simulink model "Q1"  (R2022a)
settings: Solver=FixedStepDiscrete  StartTime=0.0  StopTime=1  FixedStep=Ts  RelTol=1e-3
InitFcn:
  | Ts=50e-6;
  | 
  | % Rectifier AC side :
  | VLL_nom_R = 500e3; % V
  | Fnom_R = 60;           % Hz
  | 
  | % Inverter AC side :
  | VLL_nom_I = 345e3; % V
  | Fnom_I = 50;           % Hz
  | 
  | % DC :
  | Vdc_nom = 500e3;   % V
  | Idc_nom  = 2000;     % A
undefined symbols (not defined in the file or in its folder): D1, Delta, lagging, pulse
libraries: powerlib_extras x6, spsThreePhaseHarmonicFilterLib x6, spsImpedanceMeasurementLib x4, spsUniversalBridgeLib x4, spsThreePhaseSourceLib x2, spsSeriesRLCBranchLib x2, spsThreePhaseParallelRLCBranchLib x2, spsThreePhaseVIMeasurementLib x2, spsGroundLib x2, spsThreePhaseTransformerThreeWindingsLib x2, spsPLL3phLib x2, spsPulseGeneratorThyristor12PulseLib x2
settings Model: Creator=BhAsKaR  LastModifiedBy=ds
settings SolverCC: AlgebraicLoopSolver=TrustRegion
settings DataIOCC: SaveTime=off  ReturnWorkspaceOutputs=off
settings OptimizationCC: DefaultParameterBehavior=Inlined  EnhancedBackFolding=on  PassReuseOutputArgsAs=Individual arguments  ZeroExternalMemoryAtStartup=off  ZeroInternalMemoryAtStartup=off  OptimizeBlockOrder=speed  DifferentSizesBufferReuse=on  OptimizationCustomize=off  EfficientTunableParamExpr=on
settings DebuggingCC: ParameterTunabilityLossMsg=error  UnconnectedInputMsg=warning  UnconnectedOutputMsg=warning  SFMachineParentedDataDiag=warning
settings SFSimCC: MATLABDynamicMemAlloc=off
settings RTWCC: SystemTargetFile=ert.tlc  TemplateMakefile=ert_default_tmf
settings CodeAppCC: ForceParamTrailComments=on  IgnoreCustomStorageClasses=off  OperatorAnnotations=on  SimulinkDataObjDesc=on  SFDataObjDesc=on  InsertBlockDesc=on
settings ERTTargetCC: TargetLangStandard=C99 (ISO)  GenerateSampleERTMain=on  InlinedParameterPlacement=NonHierarchical  ERTCustomFileTemplate=example_file_process.tlc

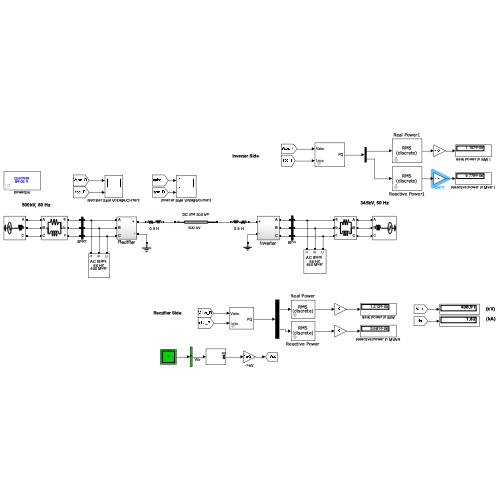
[thumbnail: Simulink's stored preview of the top-level diagram]
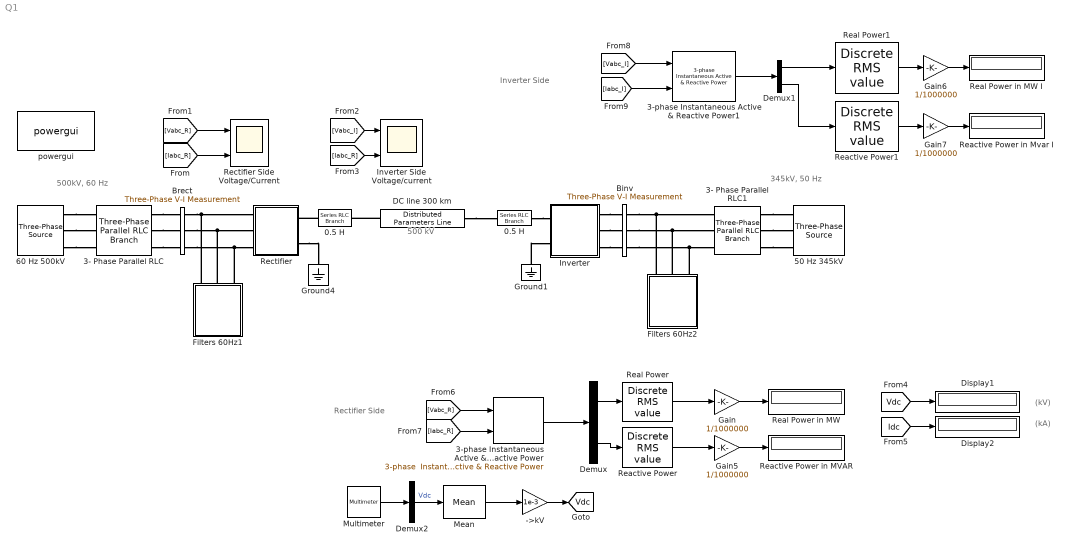
== system Q1 ==
  note: 500 kV
  note: 500kV, 60 Hz
  note: 345kV, 50 Hz
  note: (kV)
  note: Rectifier Side
  note: Inverter Side
  note: (kA)
  " 50 Hz 345kV  " : spsThreePhaseSourceLib/Three-Phase Source  InternalConnection=Yg  VoltagePhases=off  Voltage=VLL_nom_I  PhaseAngle=0  Voltage_phases=[25e3 25e3 25e3]/sqrt(3)  PhaseAngles_phases=[0 -120 +120]  Frequency=Fnom_I  NonIdealSource=on  SpecifyImpedance=off  Resistance=0  Inductance=28.0e-3  ShortCircuitLevel=0  BaseVoltage=0  XRratio=0  BusType=swing  Pref=0  Qref=0  Prefabc=[10e3, 10e3, 10e3]  Qrefabc=[0, 0, 0]  Qmin=-inf  Qmax=inf
  " 60 Hz 500kV" : spsThreePhaseSourceLib/Three-Phase Source  InternalConnection=Yg  VoltagePhases=off  Voltage=VLL_nom_R  PhaseAngle=0  Voltage_phases=[25e3 25e3 25e3]/sqrt(3)  PhaseAngles_phases=[0 -120 +120]  Frequency=Fnom_R  NonIdealSource=on  SpecifyImpedance=off  Resistance=0  Inductance=98.03e-3  ShortCircuitLevel=0  BaseVoltage=0  XRratio=0  BusType=swing  Pref=0  Qref=0  Prefabc=[10e3, 10e3, 10e3]  Qrefabc=[0, 0, 0]  Qmin=-inf  Qmax=inf
  ->kV : Gain  Gain=1e-3  SaturateOnIntegerOverflow=on  OutDataTypeStr=Inherit: Same as input  ParamDataTypeStr=Inherit: Same as input
  0.5 H : spsSeriesRLCBranchLib/Series RLC Branch  LConnTagsString=__new0  RConnTagsString=__new0  BranchType=RL  Resistance=1  Inductance=0.5  SetiL0=off  InitialCurrent=0  Capacitance=1.0  Setx0=off  InitialVoltage=0  Measurements=Branch voltage and current
  "0.5 H " : spsSeriesRLCBranchLib/Series RLC Branch  LConnTagsString=__new0  RConnTagsString=__new0  BranchType=RL  Resistance=1  Inductance=0.5  SetiL0=off  InitialCurrent=0  Capacitance=1.0  Setx0=off  InitialVoltage=0  Measurements=Branch voltage and current
  3- Phase Parallel RLC : spsThreePhaseParallelRLCBranchLib/Three-Phase Parallel RLC Branch  LConnTagsString=A|B|C  RConnTagsString=A|B|C  BranchType=RL  Resistance=26.07  Inductance=48.86e-3  Capacitance=1.0  Measurements=None
      settings: SourceProductBaseCode=PS
  3- Phase Parallel RLC1 : spsThreePhaseParallelRLCBranchLib/Three-Phase Parallel RLC Branch  LConnTagsString=A|B|C  RConnTagsString=A|B|C  BranchType=RL  Resistance=6.205  Inductance=13.96e-3  Capacitance=1.0  Measurements=None
      settings: SourceProductBaseCode=PS
  3-phase Instantaneous Active & Reactive Power : powerlib_extras/Measurements/3-phase  Instantaneous  Active & Reactive Power
      settings: SourceProductBaseCode=PS
  3-phase Instantaneous Active & Reactive Power1 : powerlib_extras/Measurements/3-phase  Instantaneous  Active & Reactive Power
      settings: SourceProductBaseCode=PS
  Binv : spsThreePhaseVIMeasurementLib/Three-Phase V-I Measurement  VoltageMeasurement=phase-to-ground  SetLabelV=on  LabelV=Vabc_I  Vpu=on  VpuLL=off  CurrentMeasurement=yes  SetLabelI=on  LabelI=Iabc_I  Ipu=on  Pbase=100e6  Vbase=345e3  OutputType=Magnitude  PhasorSimulation=off  PSBequivalent=0
  Brect : spsThreePhaseVIMeasurementLib/Three-Phase V-I Measurement  VoltageMeasurement=phase-to-ground  SetLabelV=on  LabelV=Vabc_R  Vpu=on  VpuLL=off  CurrentMeasurement=yes  SetLabelI=on  LabelI=Iabc_R  Ipu=on  Pbase=100e6  Vbase=500e3  OutputType=Magnitude  PhasorSimulation=off  PSBequivalent=0
  DC line 300 km : spsDistributedParametersLineLib/Distributed Parameters Line  Phases=1  Length=300  Frequency=60  Resistance=0.015  Inductance=0.792e-3  Capacitance=14.4e-9  x1=[-0.00105 -5.9657325618739e-12;-0.001 -5.74588371812075e-12;-0.00095 -5.52535227515782e-12;-0.0009 -5.30421024315457e-12;-0.00085 -5.08252951550024e-12;-0.0008 -4.86038184490804e-12;-0.00075 -4.63783881965118e-12;-0.0007 -4.41497183993891e-12;-0.00065 -4.19185209444034e-12;-0.0006 -3.96855053696411e-12;-0.00055 -3.74513786330158e-12;-0.0005 -3.52168448824124e-12;-0.00045 -3.29826052276211e-12;-0.0004 -3.07493575141354e-12;-0.00035 -2.85177960988905e-12;-0.0003 -2.62886116280138e-12;-0.00025 -2.40624908166623e-12;-0.0002 -2.18401162310181e-12;-0.00015 -1.96221660725129e-12;-0.0001 -1.74093139643523e-12;-5e-05 -1.52022287404077e-12]  x2=[-0.00105 -4.80956103183517e-12;-0.001 -4.57813962792348e-12;-0.00095 -4.34637866135639e-12;-0.0009 -4.11435439321598e-12;-0.00085 -3.88214286207982e-12;-0.0008 -3.64981985858362e-12;-0.00075 -3.41746090014951e-12;-0.0007 -3.18514120588852e-12;-0.00065 -2.95293567168596e-12;-0.0006 -2.72091884547773e-12;-0.00055 -2.48916490272637e-12;-0.0005 -2.2577476221045e-12;-0.00045 -2.0267403613944e-12;-0.0004 -1.79621603361121e-12;-0.00035 -1.56624708335811e-12;-0.0003 -1.33690546342109e-12;-0.00025 -1.10826261161117e-12;-0.0002 -8.80389427861601e-13;-0.00015 -6.53356251587666e-13;-0.0001 -4.27232839316443e-13;-5e-05 -2.02088342593868e-13]  x3=[-0.00105 -4.02613211172553e-14;-0.001 -3.91158507623226e-14;-0.00095 -3.79621871436524e-14;-0.0009 -3.6800712983211e-14;-0.00085 -3.56318123772384e-14;-0.0008 -3.44558706668299e-14;-0.00075 -3.32732743084192e-14;-0.0007 -3.20844107442077e-14;-0.00065 -3.08896682725833e-14;-0.0006 -2.96894359185733e-14;-0.00055 -2.84841033043753e-14;-0.0005 -2.72740605200094e-14;-0.00045 -2.60596979941367e-14;-0.0004 -2.4841406365086e-14;-0.00035 -2.36195763521336e-14;-0.0003 -2.23945986270781e-14;-0.00025 -2.1166863686155e-14;-0.0002 -1.99367617223316e-14;-0.00015 -1.87046824980275e-14;-0.0001 -1.74710152183011e-14;-5e-05 -1.62361484045448e-14]  x4=[-0.00105 -2.45317870901981e-14;-0.001 -2.38273313348991e-14;-0.00095 -2.31203473445389e-14;-0.0009 -2.241108936092e-14;-0.00085 -2.16998109680401e-14;-0.0008 -2.09867650016041e-14;-0.00075 -2.02722034591618e-14;-0.0007 -1.95563774109065e-14;-0.00065 -1.88395369111643e-14;-0.0006 -1.81219309106056e-14;-0.00055 -1.74038071692105e-14;-0.0005 -1.66854121700178e-14;-0.00045 -1.5966991033688e-14;-0.0004 -1.52487874339106e-14;-0.00035 -1.45310435136846e-14;-0.0003 -1.38139998025018e-14;-0.00025 -1.30978951344604e-14;-0.0002 -1.23829665673391e-14;-0.00015 -1.16694493026568e-14;-0.0001 -1.09575766067481e-14;-5e-05 -1.02475797328794e-14]  x5=0.00101312980412186  V1=ones(3,3)  V2=ones(3,3)  I1=ones(3,3)  I2=ones(3,3)  nHarmo=1  Measurements=Phase-to-ground voltages  Decoupling=off  VsMag0=0  VrMag0=0  VsAngle0=0  VrAngle0=0  IsMag0=0  IrMag0=0  IsAngle0=0  IrAngle0=0
      settings: AttributesFormatString=\n  SourceProductBaseCode=PS
  Demux : Demux  Outputs=2
  Demux1 : Demux  Outputs=2
  Demux2 : Demux  Outputs=[1 ]
      settings: DisplayOption=none
  Display1 : Display
      settings: Format=bank  SampleTime=Ts*20
  Display2 : Display
      settings: Format=bank  SampleTime=Ts*20
  Filters 60Hz1 : Subsystem
      mask Display: disp('AC filters \n60 Hz\n450 Mvar')
  Filters 60Hz2 : Subsystem
      mask Display: disp('AC filters \n50 Hz\n450 Mvar')
  Gain{,5..7} (4 alike) : Gain  Gain=1/1000000
  Ground1 : spsGroundLib/Ground  LConnTagsString=a
  Ground4 : spsGroundLib/Ground  LConnTagsString=a
  Inverter : Subsystem
  Inverter Side Voltage/current : Scope  NumInputPorts=2
  Mean : spsMeanLib/Mean  Freq=60  Vinit=0  Ts=Ts
  Multimeter : spsMultimeterLib/Multimeter  L=44  sel=23  yselected={}  Gain=1  OutputType=Magnitude  PlotAtSimulationStop=off  PhasorSimulation=off
  Reactive Power : powerlib_extras/Discrete Measurements/Discrete  RMS value  Freq=50  Mag_Init=0  Ts=50e-6
      settings: SourceProductBaseCode=PS
  Reactive Power in MVAR : Display
  Reactive Power in Mvar I : Display
  Reactive Power1 : powerlib_extras/Discrete Measurements/Discrete  RMS value  Freq=50  Mag_Init=0  Ts=50e-6
      settings: SourceProductBaseCode=PS
  Real Power : powerlib_extras/Discrete Measurements/Discrete  RMS value  Freq=50  Mag_Init=0  Ts=50e-6
      settings: SourceProductBaseCode=PS
  Real Power in MW : Display
  Real Power in MW I : Display
  Real Power1 : powerlib_extras/Discrete Measurements/Discrete  RMS value  Freq=50  Mag_Init=0  Ts=50e-6
      settings: SourceProductBaseCode=PS
  Rectifier : Subsystem
  Rectifier Side Voltage/Current : Scope  NumInputPorts=2
  powergui : spspowerguiLib/powergui  Priority=2  SimulationMode=Discrete  SampleTime=Ts  frequency=60  Iterations=50  frequencyindice=60  Pbase=100e6  ErrMax=1e-4  UnitsV=kV  UnitsW=MW  buscounter=0  FunctionMessages=off  echomessages=off  EnableUseOfTLC=off  CurrentSourceSwitches=off  DisableSnubberDevices=off  DisableRonSwitches=off  DisableVfSwitches=off  DisplayEquations=off  AutomaticDiscreteSolvers=off  SolverType=Tustin  Interpol=off  ExternalGateDelay=off  methode=off  Ts=0  x0status=blocks  SPID=off  SwTol=0  HookPort=off  NonlinearTolerance=1e-4  nMaxIteration=100  ContinueOnMaxIteration=off  RestoreLinks=warning  ResistiveCurrentMeasurement=off  Frange=[10:2:1500]  Ylog=off  Xlog=off  ShowGrid=on  save=on  variable=ZData  structure=Invertersignals  ZoomFFT=off  StartTime=0.4  cycles=2  DisplayStyle=1  fundamental=50  FreqAxis=off  MaxFrequency=500  frequencyindicesteady=1  RmsSteady=1  display=off
  tag scope: Vdc=global
  wires:
  [Vabc_R] -> Rectifier Side Voltage/Current/1
  [Iabc_R] -> Rectifier Side Voltage/Current/2
  [Vabc_I] -> Inverter Side Voltage/current/1
  [Iabc_R] -> Inverter Side Voltage/current/2
  Demux2/1 -> Mean/1  "Vdc"
  Multimeter/1 -> Demux2/1
  ->kV/1 -> [Vdc]
  [Idc] -> Display2/1
  Demux/2 -> Reactive Power/1
  [Vdc] -> Display1/1
  [Vabc_I] -> 3-phase Instantaneous Active & Reactive Power1/1
  Gain6/1 -> Real Power in MW I/1
  Gain/1 -> Real Power in MW/1
  3-phase Instantaneous Active & Reactive Power1/1 -> Demux1/1
  [Iabc_I] -> 3-phase Instantaneous Active & Reactive Power1/2
  Mean/1 -> ->kV/1
  [Vabc_R] -> 3-phase Instantaneous Active & Reactive Power/1
  Gain7/1 -> Reactive Power in Mvar I/1
  Demux1/2 -> Reactive Power1/1
  Reactive Power/1 -> Gain5/1
  Gain5/1 -> Reactive Power in MVAR/1
  Demux/1 -> Real Power/1
  3-phase Instantaneous Active & Reactive Power/1 -> Demux/1
  Real Power1/1 -> Gain6/1
  [Iabc_R] -> 3-phase Instantaneous Active & Reactive Power/2
  Real Power/1 -> Gain/1
  Reactive Power1/1 -> Gain7/1
  Demux1/1 -> Real Power1/1
  connections:
  Binv/LConn1 -- Filters 60Hz2/LConn1 -- 3- Phase Parallel RLC1/RConn1
  Binv/LConn2 -- Filters 60Hz2/LConn2 -- 3- Phase Parallel RLC1/RConn2
  Binv/LConn3 -- Filters 60Hz2/LConn3 -- 3- Phase Parallel RLC1/RConn3
  3- Phase Parallel RLC1/LConn1 -- " 50 Hz 345kV  "/RConn1
  " 60 Hz 500kV"/RConn2 -- 3- Phase Parallel RLC/LConn2
  " 60 Hz 500kV"/RConn3 -- 3- Phase Parallel RLC/LConn3
  Brect/RConn2 -- Filters 60Hz1/LConn2 -- Rectifier/LConn2
  Rectifier/RConn2 -- Ground4/LConn1
  3- Phase Parallel RLC1/LConn3 -- " 50 Hz 345kV  "/RConn3
  Brect/RConn1 -- Rectifier/LConn1 -- Filters 60Hz1/LConn1
  " 60 Hz 500kV"/RConn1 -- 3- Phase Parallel RLC/LConn1
  Inverter/LConn1 -- Binv/RConn1
  Brect/RConn3 -- Filters 60Hz1/LConn3 -- Rectifier/LConn3
  Inverter/LConn3 -- Binv/RConn3
  Inverter/LConn2 -- Binv/RConn2
  "0.5 H "/LConn1 -- Inverter/RConn1
  3- Phase Parallel RLC1/LConn2 -- " 50 Hz 345kV  "/RConn2
  0.5 H/LConn1 -- Rectifier/RConn1
  Ground1/LConn1 -- Inverter/RConn2
  3- Phase Parallel RLC/RConn1 -- Brect/LConn1
  3- Phase Parallel RLC/RConn2 -- Brect/LConn2
  3- Phase Parallel RLC/RConn3 -- Brect/LConn3
  DC line 300 km/LConn1 -- 0.5 H/RConn1
  DC line 300 km/RConn1 -- "0.5 H "/RConn1

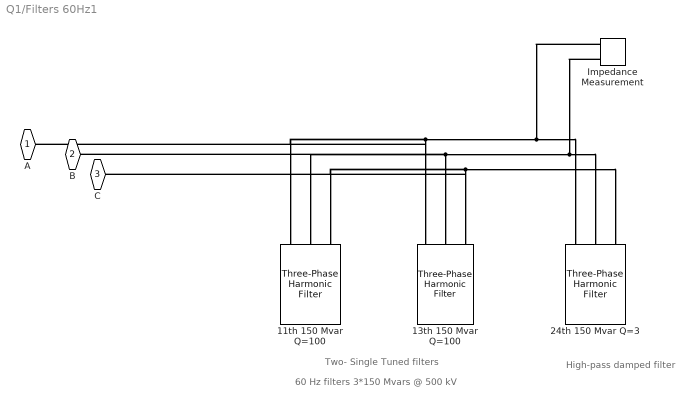
== system Q1/Filters 60Hz1 ==
  note: Two- Single Tuned filters
  note: High-pass
      | damped filter
  note: 60 Hz filters 3*150 Mvars @ 500 kV
  11th 150 Mvar Q=100 : spsThreePhaseHarmonicFilterLib/Three-Phase Harmonic Filter  LConnTagsString=A|B|C  FilterType=Single-tuned  FilterConnection=Y (grounded)  ParNom=[VLL_nom_R, Fnom_R]  Qc=0.25*(Vdc_nom*Idc_nom*0.6)  Fr=[11*Fnom_R]  Frd=[11*60 13*60]  Q=100  Measurements=None
      settings: AttributesFormatString=\n  SourceProductBaseCode=PS
  "13th 150 Mvar Q=100 " : spsThreePhaseHarmonicFilterLib/Three-Phase Harmonic Filter  LConnTagsString=A|B|C  FilterType=Single-tuned  FilterConnection=Y (grounded)  ParNom=[VLL_nom_R, Fnom_R]  Qc=0.25*(Vdc_nom*Idc_nom*0.6)  Fr=[13*Fnom_R]  Frd=[11*60 13*60]  Q=100  Measurements=None
      settings: AttributesFormatString=\n  SourceProductBaseCode=PS
  24th 150 Mvar Q=3 : spsThreePhaseHarmonicFilterLib/Three-Phase Harmonic Filter  LConnTagsString=A|B|C  FilterType=High-pass  FilterConnection=Y (grounded)  ParNom=[VLL_nom_R, Fnom_R]  Qc=0.25*(Vdc_nom*Idc_nom*0.6)  Fr=[24*Fnom_R]  Frd=[11*60 13*60]  Q=3  Measurements=None
      settings: AttributesFormatString=\n  SourceProductBaseCode=PS
  Impedance Measurement : spsImpedanceMeasurementLib/Impedance Measurement  LConnTagsString=+|-  Factor=1
      settings: SourceProductBaseCode=PS
  A : PMIOPort  Side=Left
  B : PMIOPort  Port=2  Side=Left
  C : PMIOPort  Port=3  Side=Left
  connections:
  C/RConn1 -- 11th 150 Mvar Q=100/LConn3 -- 24th 150 Mvar Q=3/LConn3 -- "13th 150 Mvar Q=100 "/LConn3
  B/RConn1 -- 11th 150 Mvar Q=100/LConn2 -- Impedance Measurement/LConn2 -- 24th 150 Mvar Q=3/LConn2 -- "13th 150 Mvar Q=100 "/LConn2
  11th 150 Mvar Q=100/LConn1 -- A/RConn1 -- Impedance Measurement/LConn1 -- 24th 150 Mvar Q=3/LConn1 -- "13th 150 Mvar Q=100 "/LConn1

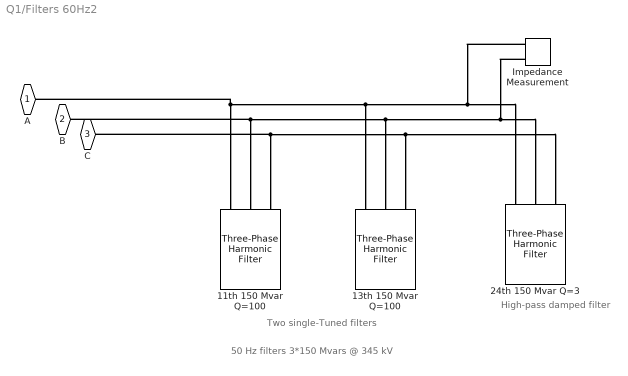
== system Q1/Filters 60Hz2 ==
  note: 50 Hz filters 3*150 Mvars @ 345 kV
  note: Two single-Tuned filters
  note: High-pass
      | damped filter
  11th 150 Mvar Q=100 : spsThreePhaseHarmonicFilterLib/Three-Phase Harmonic Filter  LConnTagsString=A|B|C  FilterType=Single-tuned  FilterConnection=Y (grounded)  ParNom=[VLL_nom_I, Fnom_I]  Qc=0.25*(Vdc_nom*Idc_nom*0.6)  Fr=[11*Fnom_I]  Frd=[11*60 13*60]  Q=100  Measurements=None
      settings: AttributesFormatString=\n  SourceProductBaseCode=PS
  "13th 150 Mvar Q=100 " : spsThreePhaseHarmonicFilterLib/Three-Phase Harmonic Filter  LConnTagsString=A|B|C  FilterType=Single-tuned  FilterConnection=Y (grounded)  ParNom=[VLL_nom_I, Fnom_I]  Qc=0.25*(Vdc_nom*Idc_nom*0.6)  Fr=[13*Fnom_I]  Frd=[11*60 13*60]  Q=100  Measurements=None
      settings: AttributesFormatString=\n  SourceProductBaseCode=PS
  24th 150 Mvar Q=3 : spsThreePhaseHarmonicFilterLib/Three-Phase Harmonic Filter  LConnTagsString=A|B|C  FilterType=High-pass  FilterConnection=Y (grounded)  ParNom=[VLL_nom_I, Fnom_I]  Qc=0.25*(Vdc_nom*Idc_nom*0.6)  Fr=[24*Fnom_I]  Frd=[11*60 13*60]  Q=3  Measurements=None
      settings: AttributesFormatString=\n  SourceProductBaseCode=PS
  Impedance Measurement : spsImpedanceMeasurementLib/Impedance Measurement  LConnTagsString=+|-  Factor=1
      settings: SourceProductBaseCode=PS
  A : PMIOPort  Side=Left
  B : PMIOPort  Port=2  Side=Left
  C : PMIOPort  Port=3  Side=Left
  connections:
  11th 150 Mvar Q=100/LConn1 -- A/RConn1 -- Impedance Measurement/LConn1 -- 24th 150 Mvar Q=3/LConn1 -- "13th 150 Mvar Q=100 "/LConn1
  11th 150 Mvar Q=100/LConn2 -- B/RConn1 -- Impedance Measurement/LConn2 -- 24th 150 Mvar Q=3/LConn2 -- "13th 150 Mvar Q=100 "/LConn2
  11th 150 Mvar Q=100/LConn3 -- C/RConn1 -- 24th 150 Mvar Q=3/LConn3 -- "13th 150 Mvar Q=100 "/LConn3

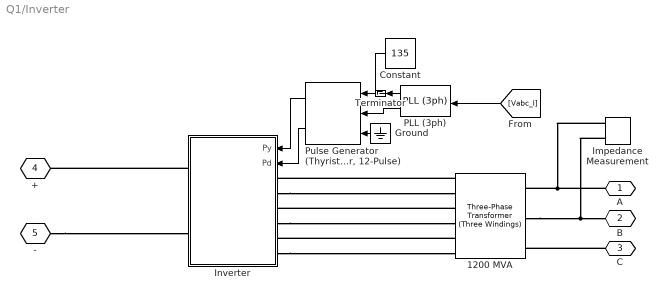
== system Q1/Inverter ==
  1200 MVA : spsThreePhaseTransformerThreeWindingsLib/Three-Phase Transformer (Three Windings)  Winding1Connection=Yg  Winding2Connection=Y  Winding3Connection=Delta (D1)  CoreType=Three single-phase transformers  SetSaturation=off  Hysteresis=off  DataFile='hysteresis'  SetInitialFlux=off  Measurements=None  UNITS=pu  NominalPower=[ 1200e6 , 50 ]  Winding1="[VLL_nom_I*0.96 0.0025  0 ]"  Winding2="[ 200e3  0.0025 0.24]"  Winding3=[ 200e3 0.0025 0.24 ]  Rm=500  Lm=500  L0=0.5  Saturation="[0 0; 0.0024 1.2; 1.0  1.45]"  InitialFluxes=[-1.10749033878531 0.564800371868647 0.542689966916658]  BreakLoop=off  DiscreteSolver=Trapezoidal iterative  DataType=off  TransfoNumber=0
      settings: AttributesFormatString=\n  SourceProductBaseCode=PS
  Constant : Constant  Value=135
  Ground : Ground
  Impedance Measurement : spsImpedanceMeasurementLib/Impedance Measurement  LConnTagsString=+|-  Factor=1
      settings: SourceProductBaseCode=PS
  Inverter : Subsystem
      mask Display: plot(0,0,100,100,[30 70 50 30 ], [60 60 40 60], [50 50], [25 40], [50 50], [ 60 75], [30 70], [40 40], [50 60 70], [40 30 30]);
  PLL (3ph) : spsPLL3phLib/PLL (3ph)  Fmin=0.75 * 50  Par_Init="[0  50]"  ParK=[180, 3200, 1]  TcD=1e-4  MaxRateChangeFreq=12  FilterCutOffFreq=25  Ts=Ts  AGC=on
  "Pulse Generator (Thyristor, 12-Pulse)" : spsPulseGeneratorThyristor12PulseLib/Pulse Generator (Thyristor, 12-Pulse)  GenType=12-pulse  Delta=D1 (lagging)  pwidth=40  Double_Pulse=on  Ts=Ts
      settings: SourceProductBaseCode=PS
  Terminator : Terminator
  A : PMIOPort  Side=Left
  B : PMIOPort  Port=2  Side=Left
  C : PMIOPort  Port=3  Side=Left
  + : PMIOPort  Port=4  Side=Right
  - : PMIOPort  Port=5  Side=Right
  wires:
  PLL (3ph)/1 -> Terminator/1
  PLL (3ph)/2 -> "Pulse Generator (Thyristor, 12-Pulse)"/2
  Constant/1 -> "Pulse Generator (Thyristor, 12-Pulse)"/1
  [Vabc_I] -> PLL (3ph)/1
  "Pulse Generator (Thyristor, 12-Pulse)"/1 -> Inverter/1(Py)
  "Pulse Generator (Thyristor, 12-Pulse)"/2 -> Inverter/2(Pd)
  Ground/1 -> "Pulse Generator (Thyristor, 12-Pulse)"/3
  connections:
  C/RConn1 -- 1200 MVA/LConn3
  A/RConn1 -- Impedance Measurement/LConn1 -- 1200 MVA/LConn1
  -/RConn1 -- Inverter/RConn2
  Inverter/LConn6 -- 1200 MVA/RConn6
  1200 MVA/RConn5 -- Inverter/LConn5
  Inverter/LConn4 -- 1200 MVA/RConn4
  1200 MVA/RConn3 -- Inverter/LConn3
  Inverter/LConn2 -- 1200 MVA/RConn2
  1200 MVA/RConn1 -- Inverter/LConn1
  1200 MVA/LConn2 -- Impedance Measurement/LConn2 -- B/RConn1
  Inverter/RConn1 -- +/RConn1

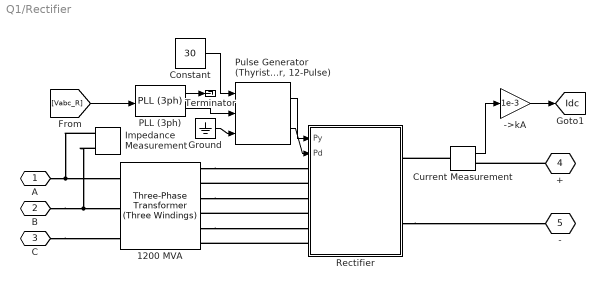
== system Q1/Rectifier ==
  ->kA : Gain  Gain=1e-3  SaturateOnIntegerOverflow=on  OutDataTypeStr=Inherit: Same as input  ParamDataTypeStr=Inherit: Same as input
  1200 MVA : spsThreePhaseTransformerThreeWindingsLib/Three-Phase Transformer (Three Windings)  Winding1Connection=Yg  Winding2Connection=Y  Winding3Connection=Delta (D1)  CoreType=Three single-phase transformers  SetSaturation=off  Hysteresis=off  DataFile='hysteresis'  SetInitialFlux=off  Measurements=None  UNITS=pu  NominalPower=[ 1200e6 , 60 ]  Winding1="[VLL_nom_R*0.9 0.0025  0 ]"  Winding2=[ 200e3 0.0025 0.24]  Winding3=[ 200e3 0.0025 0.24 ]  Rm=500  Lm=500  L0=0.5  Saturation="[0 0; 0.0024 1.2; 1.0  1.45]"  InitialFluxes=[-1.26114097729929 0.657669801639854 0.603471175659435]  BreakLoop=off  DiscreteSolver=Trapezoidal iterative  DataType=off  TransfoNumber=0
      settings: AttributesFormatString=\n  SourceProductBaseCode=PS
  Constant : Constant  Value=30
  Current Measurement : spsCurrentMeasurementLib/Current Measurement  PhasorSimulation=off  OutputType=Complex  PSBequivalent=0
  Ground : Ground
  Impedance Measurement : spsImpedanceMeasurementLib/Impedance Measurement  LConnTagsString=+|-  Factor=1
      settings: SourceProductBaseCode=PS
  PLL (3ph) : spsPLL3phLib/PLL (3ph)  Fmin=0.75*60  Par_Init="[0  60]"  ParK="[180, 3200,  1]"  TcD=1e-4  MaxRateChangeFreq=12  FilterCutOffFreq=25  Ts=Ts  AGC=on
  "Pulse Generator (Thyristor, 12-Pulse)" : spsPulseGeneratorThyristor12PulseLib/Pulse Generator (Thyristor, 12-Pulse)  GenType=12-pulse  Delta=D1 (lagging)  pwidth=40  Double_Pulse=on  Ts=Ts
      settings: SourceProductBaseCode=PS
  Rectifier : Subsystem
      mask Display: plot(0,0,100,100,[30 70 50 30 ], [40 40 60 40], [50 50], [25 40], [50 50], [ 60 75], [30 70], [60 60], [50 40 30], [60 70 70]);
  Terminator : Terminator
  A : PMIOPort  Side=Left
  B : PMIOPort  Port=2  Side=Left
  C : PMIOPort  Port=3  Side=Left
  "+ " : PMIOPort  Port=4  Side=Right
  - : PMIOPort  Port=5  Side=Right
  tag scope: Idc=global
  wires:
  "Pulse Generator (Thyristor, 12-Pulse)"/2 -> Rectifier/2(Pd)
  "Pulse Generator (Thyristor, 12-Pulse)"/1 -> Rectifier/1(Py)
  PLL (3ph)/2 -> "Pulse Generator (Thyristor, 12-Pulse)"/2
  PLL (3ph)/1 -> Terminator/1
  Ground/1 -> "Pulse Generator (Thyristor, 12-Pulse)"/3
  Constant/1 -> "Pulse Generator (Thyristor, 12-Pulse)"/1
  [Vabc_R] -> PLL (3ph)/1
  Current Measurement/1 -> ->kA/1
  ->kA/1 -> [Idc]
  connections:
  Rectifier/RConn2 -- -/RConn1
  Rectifier/LConn6 -- 1200 MVA/RConn6
  1200 MVA/RConn5 -- Rectifier/LConn5
  Rectifier/LConn4 -- 1200 MVA/RConn4
  1200 MVA/RConn3 -- Rectifier/LConn3
  Rectifier/LConn2 -- 1200 MVA/RConn2
  1200 MVA/RConn1 -- Rectifier/LConn1
  A/RConn1 -- Impedance Measurement/LConn1 -- 1200 MVA/LConn1
  B/RConn1 -- Impedance Measurement/LConn2 -- 1200 MVA/LConn2
  C/RConn1 -- 1200 MVA/LConn3
  Current Measurement/LConn1 -- Rectifier/RConn1
  "+ "/RConn1 -- Current Measurement/RConn1

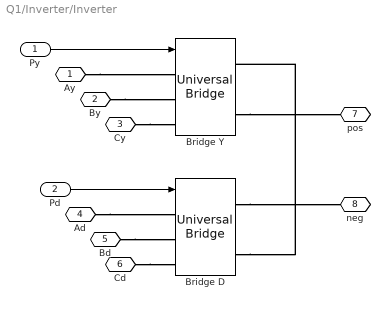
== system Q1/Inverter/Inverter ==
  Py : Inport
  Pd : Inport  Port=2
  Bridge D : spsUniversalBridgeLib/Universal Bridge  Arms=3  SnubberResistance=2000  SnubberCapacitance=0.1e-6  Device=Thyristors  Ron=1e-3  Lon=0  ForwardVoltages="[  0.8  0.8  ]"  ForwardVoltage=0  GTOparameters=[ 10e-6 , 20e-6 ]  IGBTparameters=[ 1e-6 , 2e-6 ]  Measurements=Device currents  Measurements_2=None  converterType=Rectifier
      settings: AttributesFormatString=\n
  Bridge Y : spsUniversalBridgeLib/Universal Bridge  Arms=3  SnubberResistance=2000  SnubberCapacitance=0.1e-6  Device=Thyristors  Ron=1e-3  Lon=0  ForwardVoltages="[  0.8  0.8  ]"  ForwardVoltage=0  GTOparameters=[ 10e-6 , 20e-6 ]  IGBTparameters=[ 1e-6 , 2e-6 ]  Measurements=All voltages and currents  Measurements_2=None  converterType=Rectifier
      settings: AttributesFormatString=\n
  Ay : PMIOPort  Side=Left
  By : PMIOPort  Port=2  Side=Left
  Cy : PMIOPort  Port=3  Side=Left
  Ad : PMIOPort  Port=4  Side=Left
  Bd : PMIOPort  Port=5  Side=Left
  Cd : PMIOPort  Port=6  Side=Left
  pos : PMIOPort  Port=7  Side=Right
  neg : PMIOPort  Port=8  Side=Right
  wires:
  Py/1 -> Bridge Y/1
  Pd/1 -> Bridge D/1
  connections:
  Bridge D/RConn1 -- neg/RConn1
  Bridge Y/RConn2 -- pos/RConn1
  Bridge D/RConn2 -- Bridge Y/RConn1
  Ay/RConn1 -- Bridge Y/LConn1
  By/RConn1 -- Bridge Y/LConn2
  Cy/RConn1 -- Bridge Y/LConn3
  Ad/RConn1 -- Bridge D/LConn1
  Bd/RConn1 -- Bridge D/LConn2
  Cd/RConn1 -- Bridge D/LConn3

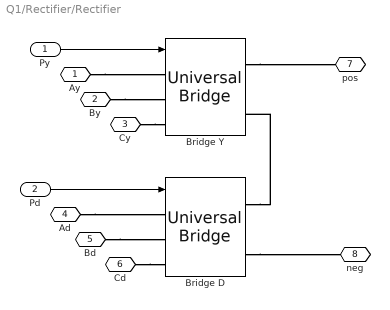
== system Q1/Rectifier/Rectifier ==
  Py : Inport
  Pd : Inport  Port=2
  Bridge D : spsUniversalBridgeLib/Universal Bridge  Arms=3  SnubberResistance=2000  SnubberCapacitance=0.1e-6  Device=Thyristors  Ron=1e-3  Lon=0  ForwardVoltages="[  0.8  0.8  ]"  ForwardVoltage=0  GTOparameters=[ 10e-6 , 20e-6 ]  IGBTparameters=[ 1e-6 , 2e-6 ]  Measurements=None  Measurements_2=None  converterType=Rectifier
      settings: AttributesFormatString=\n
  Bridge Y : spsUniversalBridgeLib/Universal Bridge  Arms=3  SnubberResistance=2000  SnubberCapacitance=0.1e-6  Device=Thyristors  Ron=1e-3  Lon=0  ForwardVoltages="[  0.8  0.8  ]"  ForwardVoltage=0  GTOparameters=[ 10e-6 , 20e-6 ]  IGBTparameters=[ 1e-6 , 2e-6 ]  Measurements=All voltages and currents  Measurements_2=None  converterType=Rectifier
      settings: AttributesFormatString=\n
  Ay : PMIOPort  Side=Left
  By : PMIOPort  Port=2  Side=Left
  Cy : PMIOPort  Port=3  Side=Left
  Ad : PMIOPort  Port=4  Side=Left
  Bd : PMIOPort  Port=5  Side=Left
  Cd : PMIOPort  Port=6  Side=Left
  pos : PMIOPort  Port=7  Side=Right
  neg : PMIOPort  Port=8  Side=Right
  wires:
  Pd/1 -> Bridge D/1
  Py/1 -> Bridge Y/1
  connections:
  Bridge D/RConn2 -- neg/RConn1
  Cd/RConn1 -- Bridge D/LConn3
  Bd/RConn1 -- Bridge D/LConn2
  Ad/RConn1 -- Bridge D/LConn1
  Cy/RConn1 -- Bridge Y/LConn3
  By/RConn1 -- Bridge Y/LConn2
  Bridge Y/RConn1 -- pos/RConn1
  Ay/RConn1 -- Bridge Y/LConn1
  Bridge D/RConn1 -- Bridge Y/RConn2
